simulink model "PID_Controller_Arm"  (R2016b)
settings: Solver=VariableStepAuto  StartTime=0.0  StopTime=200  RelTol=1e-3
values from neighbouring files (symbols this model uses):
  B = input('Enter B: ')    [HM04Nguessan.m]    (also in MTRE4010_Assignment.m = [0;KtRa/Jm]; Mtre2610_Lab7.m = im0(:,:,3))
  J = vertcat(JV,JW)    [Symbolic_Robot_Project.m]
undefined symbols (not defined in the file or in its folder): Kd, Ki, Kp, thetad
settings Model: Creator=Jacques-Ezechiel  LastModifiedBy=Jacques-Ezechiel

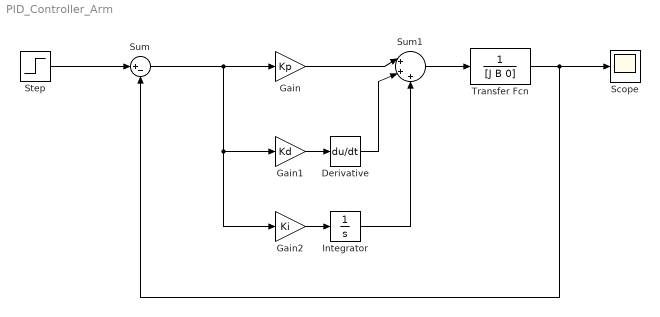
== system PID_Controller_Arm ==
  Derivative : Derivative
  Gain : Gain  Gain=Kp
  Gain1 : Gain  Gain=Kd
  Gain2 : Gain  Gain=Ki
  Integrator : Integrator
  Scope : Scope
  Step : Step  After=thetad  SampleTime=0
  Sum : Sum  Inputs=|+-
  Sum1 : Sum  Inputs=|+++
  Transfer Fcn : TransferFcn  Denominator=[J B 0]
  wires:
  Gain/1 -> Sum1/1
  Sum/1 -> Gain2/1, Gain1/1, Gain/1
  Sum1/1 -> Transfer Fcn/1
  Transfer Fcn/1 -> Sum/2, Scope/1
  Step/1 -> Sum/1
  Gain1/1 -> Derivative/1
  Derivative/1 -> Sum1/2
  Gain2/1 -> Integrator/1
  Integrator/1 -> Sum1/3
